simulink model "BeamSystem_2"  (R2020b)
settings: Solver=ode23t  StartTime=0.0  StopTime=5.5  RelTol=1e-3  AbsTol=1e-07
model workspace (MAT data in the model file):
  l = 2
  wfb = [0; 0; 0]
undefined symbols (not defined in the file): dt
libraries: lib_beam x60
settings Model: Creator=hao  LastModifiedBy=hao
settings DebuggingCC: UnconnectedInputMsg=none  UnconnectedOutputMsg=none  UnderSpecifiedDimensionMsg=warning

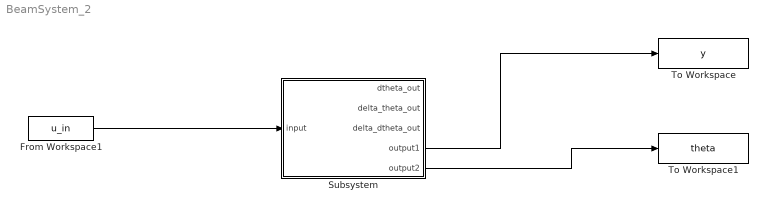
== system BeamSystem_2 ==
  From Workspace1 : FromWorkspace  VariableName=u_in  SampleTime=dt
  Subsystem : Subsystem
  To Workspace : ToWorkspace  VariableName=y  SaveFormat=Timeseries  SampleTime=dt
  To Workspace1 : ToWorkspace  VariableName=theta  SaveFormat=Timeseries  SampleTime=dt
  wires:
  Subsystem/4(output1) -> To Workspace/1
  From Workspace1/1 -> Subsystem/1(input)
  Subsystem/5(output2) -> To Workspace1/1

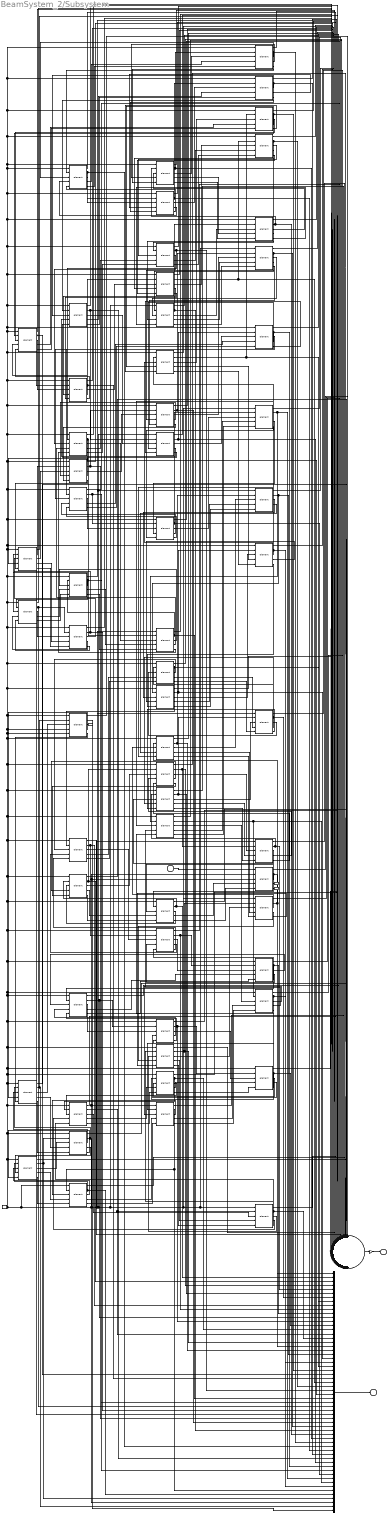
== system BeamSystem_2/Subsystem ==
  input : Inport
  bus : BusCreator  Inputs=60
  constant : Constant  Value=0
  element{1..60} (60 alike) : lib_beam/element  IA=0.005  k1=5  k2=1000  k3=10000  b=30  ElementLength=0
  gain : Gain  Gain=0.03
  sum : Sum  Inputs=60
  dtheta_out : Outport
  delta_theta_out : Outport  Port=2
  delta_dtheta_out : Outport  Port=3
  output1 : Outport  Port=4
  output2 : Outport  Port=5
  wires:
  element47/4 -> element46/4
  element57/3 -> element58/3
  element27/3 -> element28/3
  element32/1 -> sum/32
  element43/3 -> element44/3
  element46/1 -> sum/46
  element15/1 -> sum/15
  element24/3 -> element25/3
  element42/1 -> sum/42
  element17/1 -> sum/17
  element23/5 -> element22/5
  element53/3 -> element54/3
  element25/3 -> element26/3
  element47/1 -> sum/47
  element57/1 -> sum/57
  element48/3 -> element49/3
  element45/3 -> element46/3
  element11/4 -> element10/4
  element10/1 -> sum/10
  element29/5 -> element28/5
  element13/5 -> element12/5
  element46/5 -> element45/5
  element9/5 -> element8/5
  element41/4 -> element40/4
  element26/5 -> element25/5
  element6/3 -> element7/3
  element18/1 -> sum/18
  element36/3 -> element37/3
  element30/4 -> element29/4
  input/1 -> element1/1
  element10/3 -> element11/3
  element9/3 -> element10/3
  element51/3 -> element52/3
  element37/1 -> sum/37
  element2/5 -> element1/5
  element37/5 -> element36/5
  element58/4 -> element57/4
  element45/1 -> sum/45
  element3/2 -> bus/3, element4/2
  element56/4 -> element55/4
  element24/1 -> sum/24
  element40/1 -> sum/40
  element10/4 -> element9/4
  element16/5 -> element15/5
  element19/2 -> bus/19, element20/2
  element34/4 -> element33/4
  element32/4 -> element31/4
  element14/4 -> element13/4
  element40/5 -> element39/5
  element51/1 -> sum/51
  element39/1 -> sum/39
  element1/1 -> sum/1
  element36/1 -> sum/36
  element49/1 -> sum/49
  element57/4 -> element56/4
  element2/1 -> sum/2
  element24/4 -> element23/4
  element33/3 -> element34/3
  element60/3 -> dtheta_out/1
  element50/5 -> element49/5
  element30/3 -> element31/3
  element60/5 -> element59/5
  element18/3 -> element19/3
  element50/3 -> element51/3
  bus/1 -> output2/1
  element43/5 -> element42/5
  element23/4 -> element22/4
  element50/4 -> element49/4
  element38/2 -> bus/38, element39/2
  element34/1 -> sum/34
  element38/5 -> element37/5
  element51/2 -> bus/51, element52/2
  element59/3 -> element60/3
  element18/5 -> element17/5
  element6/4 -> element5/4
  element16/4 -> element15/4
  element4/1 -> sum/4
  element43/1 -> sum/43
  element23/2 -> bus/23, element24/2
  element49/2 -> bus/49, element50/2
  element36/2 -> bus/36, element37/2
  element17/5 -> element16/5
  element52/5 -> element51/5
  element8/4 -> element7/4
  element55/1 -> sum/55
  element4/3 -> element5/3
  element27/5 -> element26/5
  element7/2 -> bus/7, element8/2
  element41/1 -> sum/41
  element35/5 -> element34/5
  element10/2 -> bus/10, element11/2
  element31/4 -> element30/4
  element60/4 -> element59/4
  element12/5 -> element11/5
  element55/2 -> bus/55, element56/2
  element50/1 -> sum/50
  element39/5 -> element38/5
  element7/4 -> element6/4
  element44/4 -> element43/4
  element48/1 -> sum/48
  element13/4 -> element12/4
  element55/4 -> element54/4
  element9/1 -> sum/9
  element13/1 -> sum/13
  element44/3 -> element45/3
  element12/1 -> sum/12
  element36/4 -> element35/4
  element2/4 -> element1/4
  element30/5 -> element29/5
  element42/4 -> element41/4
  element51/4 -> element50/4
  element49/3 -> element50/3
  element54/5 -> element53/5
  element25/1 -> sum/25
  element4/4 -> element3/4
  element35/4 -> element34/4
  element56/1 -> sum/56
  element57/2 -> bus/57, element58/2
  element42/5 -> element41/5
  element15/5 -> element14/5
  element8/1 -> sum/8
  element53/1 -> sum/53
  element40/3 -> element41/3
  element25/4 -> element24/4
  element35/1 -> sum/35
  element42/3 -> element43/3
  element31/1 -> sum/31
  element52/4 -> element51/4
  element21/5 -> element20/5
  element27/2 -> bus/27, element28/2
  element4/5 -> element3/5
  element16/2 -> bus/16, element17/2
  element13/2 -> bus/13, element14/2
  element9/4 -> element8/4
  element41/5 -> element40/5
  element32/5 -> element31/5
  element19/5 -> element18/5
  element11/5 -> element10/5
  element7/3 -> element8/3
  element58/3 -> element59/3
  element28/3 -> element29/3
  element47/3 -> element48/3
  element20/1 -> sum/20
  element1/5 -> delta_dtheta_out/1
  element21/4 -> element20/4
  element54/4 -> element53/4
  gain/1 -> output1/1
  element46/3 -> element47/3
  element3/1 -> sum/3
  element59/4 -> element58/4
  element56/2 -> bus/56, element57/2
  element1/2 -> bus/1, element2/2
  element22/4 -> element21/4
  element10/5 -> element9/5
  element21/2 -> bus/21, element22/2
  element57/5 -> element56/5
  element46/2 -> bus/46, element47/2
  element56/5 -> element55/5
  element20/5 -> element19/5
  element12/2 -> bus/12, element13/2
  element29/3 -> element30/3
  element11/3 -> element12/3
  element17/2 -> bus/17, element18/2
  element2/3 -> element3/3
  element38/4 -> element37/4
  element26/2 -> bus/26, element27/2
  element37/3 -> element38/3
  element43/2 -> bus/43, element44/2
  element54/2 -> bus/54, element55/2
  sum/1 -> gain/1
  element58/1 -> sum/58
  element22/1 -> sum/22
  element38/1 -> sum/38
  element46/4 -> element45/4
  element19/1 -> sum/19
  element43/4 -> element42/4
  element32/3 -> element33/3
  element14/1 -> sum/14
  element7/5 -> element6/5
  element26/3 -> element27/3
  element60/2 -> bus/60
  element45/5 -> element44/5
  element22/5 -> element21/5
  element22/2 -> bus/22, element23/2
  element55/3 -> element56/3
  element14/3 -> element15/3
  element20/3 -> element21/3
  element3/5 -> element2/5
  element41/2 -> bus/41, element42/2
  element52/1 -> sum/52
  element29/1 -> sum/29
  element48/5 -> element47/5
  element40/2 -> bus/40, element41/2
  element58/5 -> element57/5
  element59/5 -> element58/5
  element32/2 -> bus/32, element33/2
  element27/4 -> element26/4
  element41/3 -> element42/3
  element55/5 -> element54/5
  element26/4 -> element25/4
  element53/2 -> bus/53, element54/2
  element14/5 -> element13/5
  element54/1 -> sum/54
  element5/5 -> element4/5
  element50/2 -> bus/50, element51/2
  element33/1 -> sum/33
  element27/1 -> sum/27
  element48/2 -> bus/48, element49/2
  element36/5 -> element35/5
  element40/4 -> element39/4
  element23/3 -> element24/3
  element9/2 -> bus/9, element10/2
  element34/5 -> element33/5
  element6/1 -> sum/6
  element12/3 -> element13/3
  element39/2 -> bus/39, element40/2
  element8/3 -> element9/3
  element21/3 -> element22/3
  element8/5 -> element7/5
  element58/2 -> bus/58, element59/2
  element30/2 -> bus/30, element31/2
  element5/3 -> element6/3
  element19/3 -> element20/3
  element25/2 -> bus/25, element26/2
  element29/2 -> bus/29, element30/2
  element17/4 -> element16/4
  element23/1 -> sum/23
  element18/2 -> bus/18, element19/2
  element5/4 -> element4/4
  element24/2 -> bus/24, element25/2
  element31/5 -> element30/5
  element52/2 -> bus/52, element53/2
  element11/2 -> bus/11, element12/2
  element44/2 -> bus/44, element45/2
  element15/2 -> bus/15, element16/2
  element5/2 -> bus/5, element6/2
  element59/1 -> sum/59
  element42/2 -> bus/42, element43/2
  element12/4 -> element11/4
  element2/2 -> bus/2, element3/2
  element33/5 -> element32/5
  element52/3 -> element53/3
  element49/5 -> element48/5
  element1/3 -> element2/3
  element53/5 -> element52/5
  element1/4 -> delta_theta_out/1
  element20/4 -> element19/4
  element22/3 -> element23/3
  element11/1 -> sum/11
  element28/1 -> sum/28
  element38/3 -> element39/3
  element16/3 -> element17/3
  element8/2 -> bus/8, element9/2
  element48/4 -> element47/4
  element28/4 -> element27/4
  element39/4 -> element38/4
  element33/2 -> bus/33, element34/2
  element14/2 -> bus/14, element15/2
  element39/3 -> element40/3
  element28/2 -> bus/28, element29/2
  element45/4 -> element44/4
  element44/5 -> element43/5
  element47/2 -> bus/47, element48/2
  element56/3 -> element57/3
  element54/3 -> element55/3
  element15/3 -> element16/3
  element5/1 -> sum/5
  element37/4 -> element36/4
  element3/4 -> element2/4
  element18/4 -> element17/4
  element53/4 -> element52/4
  element49/4 -> element48/4
  element4/2 -> bus/4, element5/2
  element31/3 -> element32/3
  element26/1 -> sum/26
  element28/5 -> element27/5
  element13/3 -> element14/3
  element31/2 -> bus/31, element32/2
  element45/2 -> bus/45, element46/2
  element30/1 -> sum/30
  element15/4 -> element14/4
  element34/3 -> element35/3
  element29/4 -> element28/4
  element24/5 -> element23/5
  element37/2 -> bus/37, element38/2
  element3/3 -> element4/3
  element51/5 -> element50/5
  element7/1 -> sum/7
  element35/2 -> bus/35, element36/2
  element6/2 -> bus/6, element7/2
  element6/5 -> element5/5
  constant/1 -> element17/1, element39/1, element52/1, element19/1, element40/1, element21/1, element48/1, element32/1, element7/1, element5/1, element1/2, element1/3, element55/1, element56/1, element43/1, element46/1, element25/1, element29/1, element42/1, element44/1, element45/1, element41/1, element30/1, element28/1, element47/1, element49/1, element26/1, element24/1, element27/1, element38/1, element31/1, element37/1, element50/1, element51/1, element23/1, element36/1, element33/1, element34/1, element35/1, element8/1, element22/1, element60/1, element60/4, element60/5, element20/1, element4/1, element6/1, element53/1, element9/1, element3/1, element2/1, element10/1, element11/1, element54/1, element12/1, element13/1, element18/1, element14/1, element15/1, element59/1, element16/1, element58/1, element57/1
  element35/3 -> element36/3
  element21/1 -> sum/21
  element19/4 -> element18/4
  element33/4 -> element32/4
  element16/1 -> sum/16
  element44/1 -> sum/44
  element59/2 -> bus/59, element60/2
  element25/5 -> element24/5
  element20/2 -> bus/20, element21/2
  element34/2 -> bus/34, element35/2
  element47/5 -> element46/5
  element17/3 -> element18/3
  element60/1 -> sum/60
